simulink model "Heli_Controller_Testing"  (R2024a)
settings: Solver=ode1  StartTime=0.0  StopTime=80  FixedStep=0.01  RelTol=1e-3  EnableMultiTasking=on
values from neighbouring files (symbols this model uses):
  D2R = pi/180.0    (= 0.0174532925199)    [Heli_Setup.m]
  ELEV_SLF = 24.25    [Heli_Setup.m]
  K_CABLE = 5    [Heli_Setup.m]
  K_DAQ = 10    [Heli_Setup.m]
  Kd = 0    [Heli_Setup.m]
  Kdt = 0    [Heli_Setup.m]
  KE_C2D = -360/4096    (= -0.087890625)    [Heli_Setup.m]
  Ki = 0    [Heli_Setup.m]
  Kit = 0    [Heli_Setup.m]
  Kp = 0    [Heli_Setup.m]
  Kpt = 0    [Heli_Setup.m]
  R2D = 180/pi    (= 57.2957795131)    [Heli_Setup.m]
  TRAV_SS = 90    [Heli_Setup.m]
  U_MAX = (VSUM_MAX - Vsum)*0.5    (= 15.4767485)    [Heli_Setup.m]
  VSUM_MAX = 36    [Heli_Setup.m]
undefined symbols (not defined in the file or in its folder): HIL, qc_get_step_size
libraries: quarc_library x5
settings Model: SimulationMode=external  ExtModeTrigDuration=10000  Creator=Admin  LastModifiedBy=danielmielnik
settings SolverCC: AlgebraicLoopSolver=TrustRegion  PositivePriorityOrder=on
settings DataIOCC: SaveFormat=StructureWithTime  ReturnWorkspaceOutputs=off
settings OptimizationCC: ExpressionDepthLimit=2147483647  LifeSpan=inf
settings DebuggingCC: UnderspecifiedInitializationDetection=Classic  MergeDetectMultiDrivingBlocksExec=none  SolverPrmCheckMsg=warning  UnconnectedInputMsg=warning  UnconnectedOutputMsg=warning  UnconnectedLineMsg=warning  AllowSymbolicDim=off  StateNameClashWarn=warning  SFUnexpectedBacktrackingDiag=warning  SFNoUnconditionalDefaultTransitionDiag=warning  SFExecutionAtInitializationDiag=none  ArithmeticOperatorsInVariantConditions=warning
settings HardwareCC: ProdBitPerPointer=32  ProdBitPerSizeT=32  ProdBitPerPtrDiffT=32  ProdLargestAtomicFloat=None  ProdIntDivRoundTo=Undefined  ProdEndianess=Unspecified  ProdWordSize=32  ProdHWDeviceType=32-bit Generic
settings ModelReferenceCC: EnableRefExpFcnMdlSchedulingChecks=on  PropagateSignalLabelsOutOfModel=off
settings SFSimCC: SimUseLocalCustomCode=off  CustomCodeUndefinedFunction=UseInterfaceOnly
settings RTWCC: Description=QUARC Win64 Target  SystemTargetFile=quarc_win64.tlc  TemplateMakefile=quarc_default_tmf  RTWUseLocalCustomCode=off  GPUComputeCapability=3.5
settings CodeAppCC: StateflowObjectComments=on
settings STFCustomTargetCC: TargetPreCompLibLocation=C:\PROGRA~3\QUARC\lib\2015b\win64\release  TargetLangStandard=C89/C90 (ANSI)  ConcurrentExecutionCompliant=on  CombineOutputUpdateFcns=on  CPPClassGenCompliant=on  GRTInterface=off  UseToolchainInfoCompliant=off  SystemTargetFile=quarc_win64.tlc
settings GRTTargetCC: TargetPreCompLibLocation=C:\PROGRA~3\QUARC\lib\2015b\win64\release  TargetLangStandard=C89/C90 (ANSI)  ParMdlRefBuildCompliant=off  CompOptLevelCompliant=off  MatFileLogging=off  UseToolchainInfoCompliant=off  ExtMode=on  ExtModeMexFile=quarc_comm
settings ConfigComp: CovMetricSettings=dw  CovSaveCumulativeToWorkspaceVar=on  CovSaveSingleToWorkspaceVar=on  CovExternalEMLEnable=off

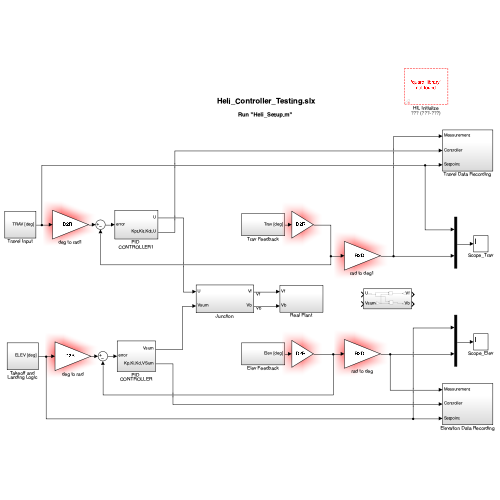
[thumbnail: Simulink's stored preview of the top-level diagram]
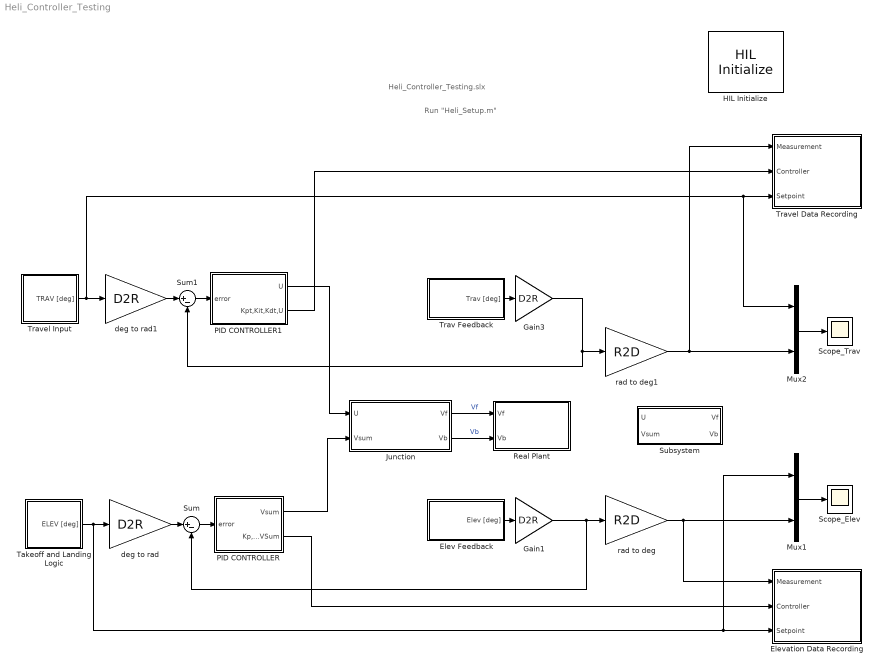
== system Heli_Controller_Testing ==
  note: Run "Heli_Setup.m"
  note: Heli_Controller_Testing.slx
  Elev Feedback : Subsystem
  Elevation Data Recording : Subsystem
  Gain1 : Gain  Gain=D2R
  Gain3 : Gain  Gain=D2R
  HIL Initialize : quarc_library/Data Acquisition/Generic/Configuration/HIL Initialize  Priority=-99  object_name=HIL-1  board_type=q4  board_number=0  board_options=""  exclusive=off  active=off  hardware_clocks=[0:1]  clock_modes=[0 0]  initial_clock_frequencies=[]  set_clock_params_at_start=on  set_clock_params_at_switch_in=off  set_clock_frequencies_at_start=off  set_clock_frequencies_at_switch_in=off  analog_input_channels=[0:3]  analog_input_maximums=10  analog_input_minimums=-10  set_analog_input_params_at_start=off  set_analog_input_params_at_switch_in=off  analog_output_channels=[0:3]  analog_output_maximums=[10]  analog_output_minimums=[-10]  initial_analog_outputs=[0]  final_analog_outputs=[0]  watchdog_analog_outputs=0  set_analog_output_params_at_start=on  set_analog_output_params_at_switch_in=off  set_analog_outputs_at_start=on  set_analog_outputs_at_switch_in=off  set_analog_outputs_at_terminate=on  set_analog_outputs_at_switch_out=off  set_analog_outputs_on_watchdog=off  digital_input_channels=[]  digital_output_channels=[]  digital_output_configuration=[]  initial_digital_outputs=[1]  final_digital_outputs=[1]  watchdog_digital_outputs=[2]  set_digital_output_params_at_start=off  set_digital_output_params_at_switch_in=off  set_digital_outputs_at_start=on  set_digital_outputs_at_switch_in=off  set_digital_outputs_at_terminate=on  set_digital_outputs_at_switch_out=off  set_digital_outputs_on_watchdog=off  encoder_channels=[0:3]  quadrature=[4]  encoder_filter_frequency=(1/60e-9)/1  initial_encoder_counts=[0]  set_encoder_params_at_start=on  set_encoder_params_at_switch_in=off  set_encoder_counts_at_start=on  set_encoder_counts_at_switch_in=off  pwm_channels=[]  pwm_modes=[0]  pwm_frequency=(1/60e-9)/1024  pwm_configuration=[]  pwm_alignment=[]  pwm_polarity=[]  pwm_leading_deadband=[]  pwm_trailing_deadband=[]  initial_pwm_outputs=[0]  final_pwm_outputs=[0]  watchdog_pwm_outputs=[]  set_pwm_params_at_start=on  set_pwm_params_at_switch_in=off  set_pwm_outputs_at_start=on  set_pwm_outputs_at_switch_in=off  set_pwm_outputs_at_terminate=on  set_pwm_outputs_at_switch_out=off  set_pwm_outputs_on_watchdog=off  other_output_channels=[]  initial_other_outputs=[]  final_other_outputs=[]  watchdog_other_outputs=[]  set_other_outputs_at_start=off  set_other_outputs_at_switch_in=off  set_other_outputs_at_terminate=off  set_other_outputs_at_switch_out=off  set_other_outputs_on_watchdog=off
  Junction : Subsystem
  Mux1 : Mux  Inputs=2
  Mux2 : Mux  Inputs=2
  PID CONTROLLER : Subsystem
  PID CONTROLLER1 : Subsystem
  Real Plant : Subsystem
  Scope_Elev : Scope
  Scope_Trav : Scope
  Subsystem : Subsystem
  Sum : Sum  Inputs=|+-
  Sum1 : Sum  Inputs=|+-
  Takeoff and Landing Logic : Subsystem
  Trav Feedback : Subsystem
  Travel Data Recording : Subsystem
  Travel Input : Subsystem
  deg to rad : Gain  Gain=D2R
  deg to rad1 : Gain  Gain=D2R
  rad to deg : Gain  Gain=R2D
  rad to deg1 : Gain  Gain=R2D
  wires:
  Sum/1 -> PID CONTROLLER/1(error)
  rad to deg/1 -> Mux1/2, Elevation Data Recording/1(Measurement)
  deg to rad/1 -> Sum/1
  Takeoff and Landing Logic/1(ELEV [deg]) -> Elevation Data Recording/3(Setpoint), Mux1/1, deg to rad/1
  Mux1/1 -> Scope_Elev/1
  PID CONTROLLER/2(Kp,Ki,Kd,VSum) -> Elevation Data Recording/2(Controller)
  Elev Feedback/1(Elev [deg]) -> Gain1/1
  deg to rad1/1 -> Sum1/1
  Sum1/1 -> PID CONTROLLER1/1(error)
  PID CONTROLLER1/2(Kpt,Kit,Kdt,U) -> Travel Data Recording/2(Controller)
  Travel Input/1(TRAV [deg]) -> deg to rad1/1, Mux2/1, Travel Data Recording/3(Setpoint)
  Trav Feedback/1(Trav [deg]) -> Gain3/1
  Mux2/1 -> Scope_Trav/1
  rad to deg1/1 -> Travel Data Recording/1(Measurement), Mux2/2
  Gain3/1 -> Sum1/2, rad to deg1/1
  Gain1/1 -> Sum/2, rad to deg/1
  Junction/2(Vb) -> Real Plant/2(Vb)  "Vb"
  PID CONTROLLER1/1(U) -> Junction/1(U)
  PID CONTROLLER/1(Vsum) -> Junction/2(Vsum)
  Junction/1(Vf) -> Real Plant/1(Vf)  "Vf"

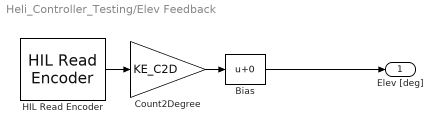
== system Heli_Controller_Testing/Elev Feedback ==
  Bias : Bias  SaturateOnIntegerOverflow=off
  Count2Degree : Gain  Gain=KE_C2D
  HIL Read Encoder : quarc_library/Data Acquisition/Generic/Immediate I//O/HIL Read Encoder  object_name=HIL-1  channels=3  sample_time=qc_get_step_size  active=on  vector_output=off  data_type_mode=Inherit via back propagation  data_type=double
  Elev [deg] : Outport
  wires:
  Count2Degree/1 -> Bias/1
  Bias/1 -> Elev [deg]/1
  HIL Read Encoder/1 -> Count2Degree/1

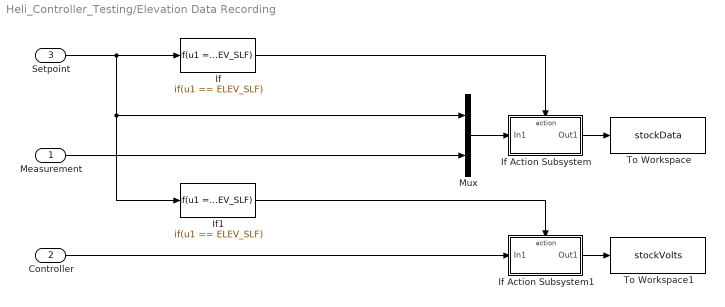
== system Heli_Controller_Testing/Elevation Data Recording ==
  Measurement : Inport
  Controller : Inport  Port=2
  Setpoint : Inport  Port=3
  If : If  IfExpression=u1 == ELEV_SLF  ShowElse=off
  If Action Subsystem : Subsystem  TreatAsAtomicUnit=on
  If Action Subsystem1 : Subsystem  TreatAsAtomicUnit=on
  If1 : If  IfExpression=u1 == ELEV_SLF  ShowElse=off
  Mux : Mux  Inputs=2
  To Workspace : ToWorkspace  VariableName=stockData  SaveFormat=Structure With Time  SampleTime=-1
  To Workspace1 : ToWorkspace  VariableName=stockVolts  SaveFormat=Structure With Time  SampleTime=-1
  wires:
  Mux/1 -> If Action Subsystem/1(In1)
  If Action Subsystem/1(Out1) -> To Workspace/1
  If/1 -> If Action Subsystem/Action
  Setpoint/1 -> If1/1, Mux/1, If/1
  If1/1 -> If Action Subsystem1/Action
  Controller/1 -> If Action Subsystem1/1(In1)
  If Action Subsystem1/1(Out1) -> To Workspace1/1
  Measurement/1 -> Mux/2

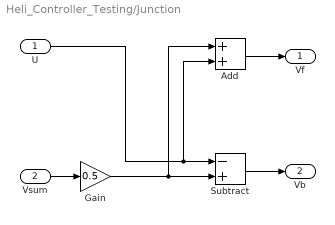
== system Heli_Controller_Testing/Junction ==
  U : Inport
  Vsum : Inport  Port=2
  Add : Sum
  Gain : Gain  Gain=0.5
  Subtract : Sum  Inputs=-+
  Vf : Outport
  Vb : Outport  Port=2
  wires:
  Add/1 -> Vf/1
  Subtract/1 -> Vb/1
  Vsum/1 -> Gain/1
  Gain/1 -> Add/1, Subtract/2
  U/1 -> Add/2, Subtract/1

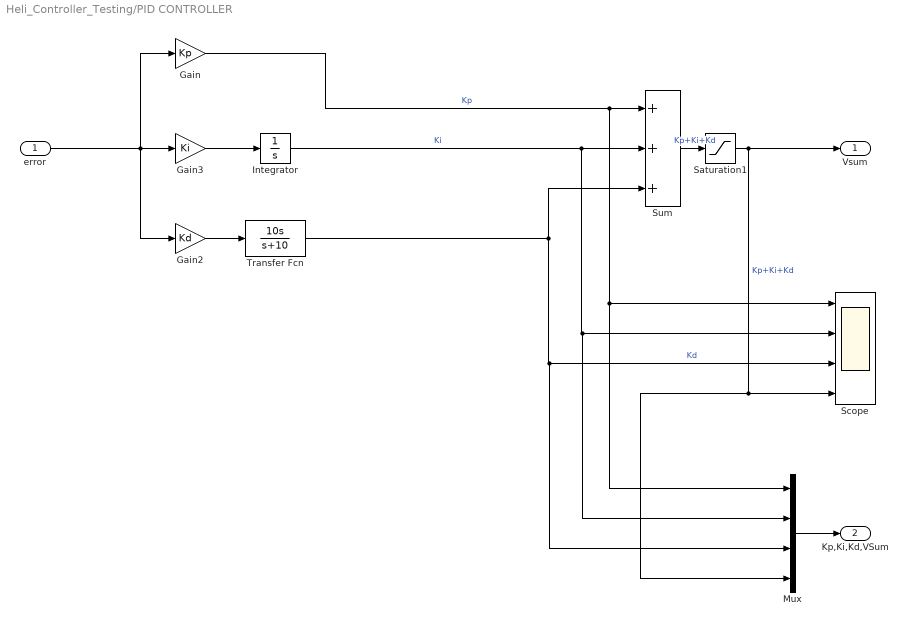
== system Heli_Controller_Testing/PID CONTROLLER ==
  error : Inport
  Gain : Gain  Gain=Kp
  Gain2 : Gain  Gain=Kd
  Gain3 : Gain  Gain=Ki
  Integrator : Integrator
  Mux : Mux
  Saturation1 : Saturate  UpperLimit=VSUM_MAX  LowerLimit=-VSUM_MAX
  Scope : Scope  NumInputPorts=4
  Sum : Sum  Inputs=+++
  Transfer Fcn : TransferFcn  Numerator=[10 0]  Denominator=[1 10]
  Vsum : Outport
  Kp,Ki,Kd,VSum : Outport  Port=2
  wires:
  Gain3/1 -> Integrator/1
  Gain/1 -> Scope/1, Mux/1, Sum/1  "Kp"
  Gain2/1 -> Transfer Fcn/1
  Sum/1 -> Saturation1/1  "Kp+Ki+Kd"
  Transfer Fcn/1 -> Mux/3, Scope/3, Sum/3  "Kd"
  Integrator/1 -> Mux/2, Scope/2, Sum/2  "Ki"
  error/1 -> Gain3/1, Gain2/1, Gain/1
  Mux/1 -> Kp,Ki,Kd,VSum/1
  Saturation1/1 -> Vsum/1, Mux/4, Scope/4  "Kp+Ki+Kd"

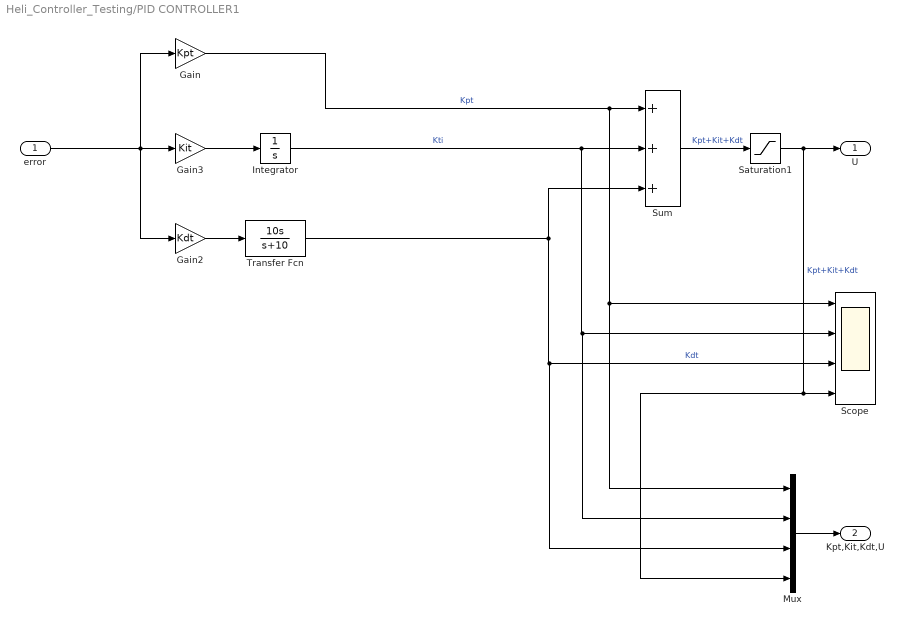
== system Heli_Controller_Testing/PID CONTROLLER1 ==
  error : Inport
  Gain : Gain  Gain=Kpt
  Gain2 : Gain  Gain=Kdt
  Gain3 : Gain  Gain=Kit
  Integrator : Integrator
  Mux : Mux
  Saturation1 : Saturate  UpperLimit=U_MAX  LowerLimit=-U_MAX
  Scope : Scope  NumInputPorts=4
  Sum : Sum  Inputs=+++
  Transfer Fcn : TransferFcn  Numerator=[10 0]  Denominator=[1 10]
  U : Outport
  Kpt,Kit,Kdt,U : Outport  Port=2
  wires:
  Gain3/1 -> Integrator/1
  Gain/1 -> Scope/1, Mux/1, Sum/1  "Kpt"
  Gain2/1 -> Transfer Fcn/1
  Sum/1 -> Saturation1/1  "Kpt+Kit+Kdt"
  Transfer Fcn/1 -> Mux/3, Scope/3, Sum/3  "Kdt"
  Integrator/1 -> Mux/2, Scope/2, Sum/2  "Kti"
  error/1 -> Gain3/1, Gain2/1, Gain/1
  Mux/1 -> Kpt,Kit,Kdt,U/1
  Saturation1/1 -> U/1, Mux/4, Scope/4  "Kpt+Kit+Kdt"

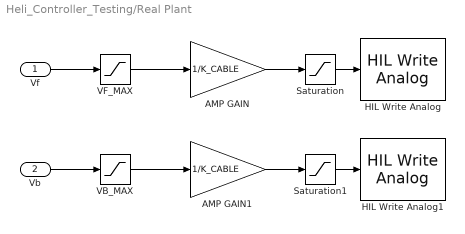
== system Heli_Controller_Testing/Real Plant ==
  Vf : Inport
  Vb : Inport  Port=2
  AMP GAIN : Gain  Gain=1/K_CABLE
  AMP GAIN1 : Gain  Gain=1/K_CABLE
  HIL Write Analog : quarc_library/Data Acquisition/Generic/Immediate I//O/HIL Write Analog  object_name=HIL-1  channels=3  sample_time=-1  active=off  vector_input=off
  HIL Write Analog1 : quarc_library/Data Acquisition/Generic/Immediate I//O/HIL Write Analog  object_name=HIL-1  channels=2  sample_time=-1  active=off  vector_input=off
  Saturation : Saturate  UpperLimit=K_DAQ*0.5  LowerLimit=-K_DAQ*0.5
  Saturation1 : Saturate  UpperLimit=K_DAQ*0.5  LowerLimit=-K_DAQ*0.5
  VB_MAX : Saturate  UpperLimit=VSUM_MAX*0.5  LowerLimit=-VSUM_MAX*0.5
  VF_MAX : Saturate  UpperLimit=VSUM_MAX*0.5  LowerLimit=-VSUM_MAX*0.5  LinearizeAsGain=off
  wires:
  Vf/1 -> VF_MAX/1
  AMP GAIN/1 -> Saturation/1
  Saturation/1 -> HIL Write Analog/1
  Saturation1/1 -> HIL Write Analog1/1
  VF_MAX/1 -> AMP GAIN/1
  Vb/1 -> VB_MAX/1
  VB_MAX/1 -> AMP GAIN1/1
  AMP GAIN1/1 -> Saturation1/1

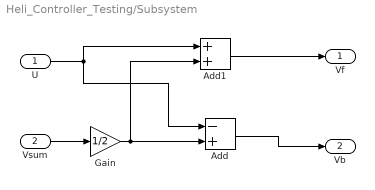
== system Heli_Controller_Testing/Subsystem ==
  U : Inport
  Vsum : Inport  Port=2
  Add : Sum  Inputs=-+
  Add1 : Sum
  Gain : Gain  Gain=1/2
  Vf : Outport
  Vb : Outport  Port=2
  wires:
  Add1/1 -> Vf/1
  Vsum/1 -> Gain/1
  U/1 -> Add/1, Add1/1
  Gain/1 -> Add1/2, Add/2
  Add/1 -> Vb/1

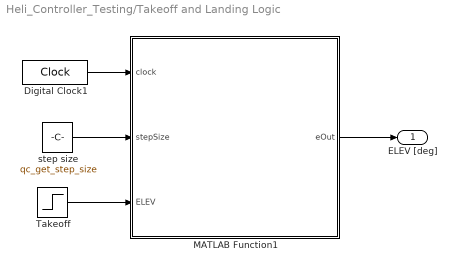
== system Heli_Controller_Testing/Takeoff and Landing Logic ==
  Digital Clock1 : DigitalClock  SampleTime=qc_get_step_size
  MATLAB Function1 : MATLAB Function  TreatAsAtomicUnit=on
  Takeoff : Step  After=ELEV_SLF  SampleTime=0
  step size : Constant  Value=qc_get_step_size
  ELEV [deg] : Outport
  wires:
  Takeoff/1 -> MATLAB Function1/3(ELEV)
  Digital Clock1/1 -> MATLAB Function1/1(clock)
  step size/1 -> MATLAB Function1/2(stepSize)
  MATLAB Function1/1(eOut) -> ELEV [deg]/1

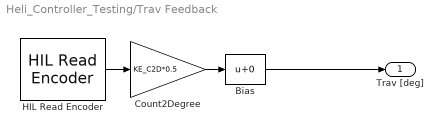
== system Heli_Controller_Testing/Trav Feedback ==
  Bias : Bias  SaturateOnIntegerOverflow=off
  Count2Degree : Gain  Gain=KE_C2D*0.5
  HIL Read Encoder : quarc_library/Data Acquisition/Generic/Immediate I//O/HIL Read Encoder  object_name=HIL-1  channels=1  sample_time=qc_get_step_size  active=on  vector_output=off  data_type_mode=Inherit via back propagation  data_type=double
  Trav [deg] : Outport
  wires:
  Count2Degree/1 -> Bias/1
  Bias/1 -> Trav [deg]/1
  HIL Read Encoder/1 -> Count2Degree/1

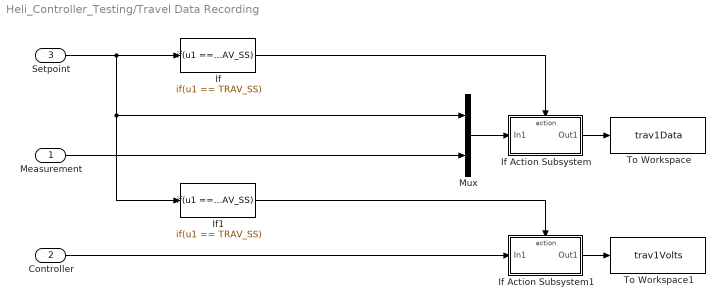
== system Heli_Controller_Testing/Travel Data Recording ==
  Measurement : Inport
  Controller : Inport  Port=2
  Setpoint : Inport  Port=3
  If : If  IfExpression=u1 == TRAV_SS  ShowElse=off
  If Action Subsystem : Subsystem  TreatAsAtomicUnit=on
  If Action Subsystem1 : Subsystem  TreatAsAtomicUnit=on
  If1 : If  IfExpression=u1 == TRAV_SS  ShowElse=off
  Mux : Mux  Inputs=2
  To Workspace : ToWorkspace  VariableName=trav1Data  SaveFormat=Structure With Time  SampleTime=-1
  To Workspace1 : ToWorkspace  VariableName=trav1Volts  SaveFormat=Structure With Time  SampleTime=-1
  wires:
  Mux/1 -> If Action Subsystem/1(In1)
  If Action Subsystem/1(Out1) -> To Workspace/1
  If/1 -> If Action Subsystem/Action
  Setpoint/1 -> If1/1, Mux/1, If/1
  If1/1 -> If Action Subsystem1/Action
  Controller/1 -> If Action Subsystem1/1(In1)
  If Action Subsystem1/1(Out1) -> To Workspace1/1
  Measurement/1 -> Mux/2

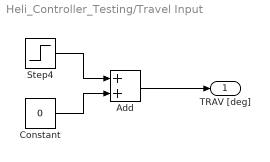
== system Heli_Controller_Testing/Travel Input ==
  Add : Sum
  Constant : Constant  Value=0
  Step4 : Step  Time=20  After=TRAV_SS  SampleTime=0
  TRAV [deg] : Outport
  wires:
  Constant/1 -> Add/2
  Add/1 -> TRAV [deg]/1
  Step4/1 -> Add/1

== system Heli_Controller_Testing/Elevation Data Recording/If Action Subsystem ==
  In1 : Inport
  Action Port : ActionPort  InitializeStates=reset  ActionPortLabel=if { }
  Out1 : Outport
  wires:
  In1/1 -> Out1/1

== system Heli_Controller_Testing/Elevation Data Recording/If Action Subsystem1 ==
  In1 : Inport
  Action Port : ActionPort  InitializeStates=reset  ActionPortLabel=if { }
  Out1 : Outport
  wires:
  In1/1 -> Out1/1

== system Heli_Controller_Testing/Travel Data Recording/If Action Subsystem ==
  In1 : Inport
  Action Port : ActionPort  InitializeStates=reset  ActionPortLabel=if { }
  Out1 : Outport
  wires:
  In1/1 -> Out1/1

== system Heli_Controller_Testing/Travel Data Recording/If Action Subsystem1 ==
  In1 : Inport
  Action Port : ActionPort  InitializeStates=reset  ActionPortLabel=if { }
  Out1 : Outport
  wires:
  In1/1 -> Out1/1

== matlab function Heli_Controller_Testing/Takeoff and Landing Logic/MATLAB Function1 ==
  data: clock input; stepSize input; eOut output; ELEV input
function eOut = fcn(clock,stepSize,ELEV)
%#codegen

persistent elevOut;
if isempty(elevOut)
    elevOut = 0;
end    

if(clock < 55)
    elevOut = ELEV;
else
    elevOut = elevOut - ELEV/clock*stepSize*2;
end
eOut = elevOut;
